simulink model "modelrevfinalPOSITIONcontrol"  (R2017b)
settings: Solver=VariableStepAuto  StartTime=0.0  StopTime=4  RelTol=1e-3
values from neighbouring files (symbols this model uses):
  D_d = 0.0034    [modelrevfinalparameters.mat]
  D_m = 0.00526687727141    [modelrevfinalparameters.mat]
  GR = 0.0526315789474    [modelrevfinalparameters.mat]
  J_l = 0.0012    [modelrevfinalparameters.mat]
  J_m = 0.0001    [modelrevfinalparameters.mat]
  k_e = 0.0064    [modelrevfinalparameters.mat]
  k_t = 0.0071    [modelrevfinalparameters.mat]
  L_a = 0.00487030359254    [modelrevfinalparameters.mat]
  m_d = 0.333333333333    [modelrevfinalparameters.mat]
  m_l = 0.333333333333    [modelrevfinalparameters.mat]
  R_a = 2.4    [modelrevfinalparameters.mat]
libraries: simulink x1
settings Model: Creator=Yusuf  LastModifiedBy=Yusuf

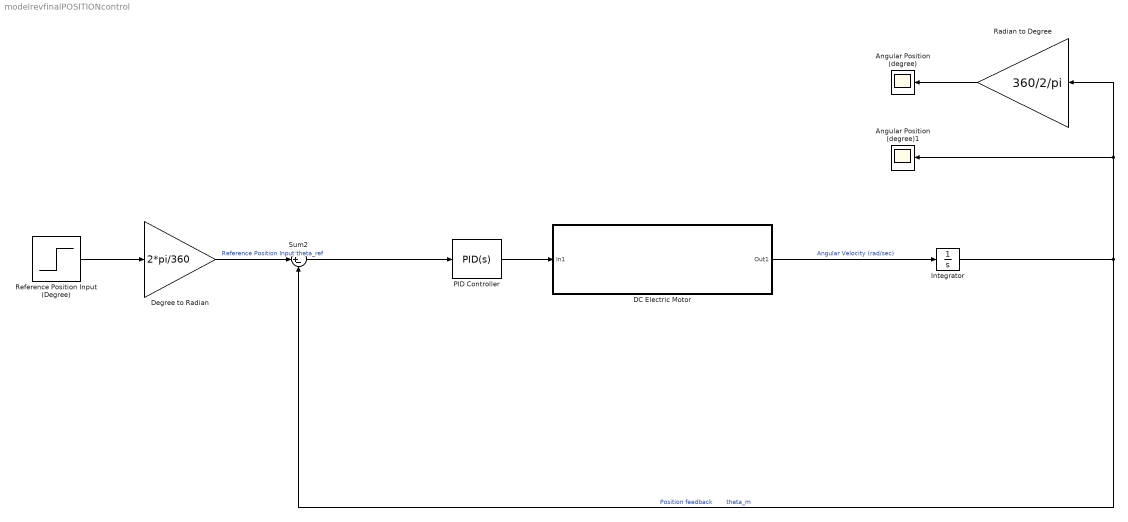
== system modelrevfinalPOSITIONcontrol ==
  Angular Position (degree) : Scope
  Angular Position (degree)1 : Scope
  DC Electric Motor : Subsystem
  Degree to Radian : Gain  Gain=2*pi/360
  Integrator : Integrator
  PID Controller : simulink/Continuous/PID Controller  Controller=PID  TimeDomain=Continuous-time  SampleTime=-1  IntegratorMethod=Forward Euler  FilterMethod=Forward Euler  Form=Parallel  UseFilter=on  ControllerParametersSource=internal  P=1.5  I=0  D=0  N=100  InitialConditionSource=internal  InitialConditionForIntegrator=0  InitialConditionForFilter=0  ExternalReset=none  LimitOutput=off  UpperSaturationLimit=inf  LowerSaturationLimit=-inf  LinearizeAsGain=on  AntiWindupMode=none  Kb=1  TrackingMode=off  Kt=1  PParamMin=[]  PParamMax=[]  IParamMin=[]  IParamMax=[]  DParamMin=[]  DParamMax=[]  NParamMin=[]  NParamMax=[]  KbParamMin=[]  KbParamMax=[]  KtParamMin=[]  KtParamMax=[]  POutMin=[]  POutMax=[]  IOutMin=[]  IOutMax=[]  DOutMin=[]  DOutMax=[]  NOutMin=[]  NOutMax=[]  KbOutMin=[]  KbOutMax=[]  KtOutMin=[]  KtOutMax=[]  IntegratorOutMin=[]  IntegratorOutMax=[]  FilterOutMin=[]  FilterOutMax=[]  SumOutMin=[]  SumOutMax=[]  SumI1OutMin=[]  SumI1OutMax=[]  SumI2OutMin=[]  SumI2OutMax=[]  SumI3OutMin=[]  SumI3OutMax=[]  SumDOutMin=[]  SumDOutMax=[]  SaturationOutMin=[]  SaturationOutMax=[]  IntegratorContinuousStateAttributes=''  IntegratorStateMustResolveToSignalObject=off  IntegratorRTWStateStorageClass=Auto  FilterContinuousStateAttributes=''  FilterStateMustResolveToSignalObject=off  FilterRTWStateStorageClass=Auto  DifferentiatorICPrevScaledInput=0  DifferentiatorOutMin=[]  DifferentiatorOutMax=[]  InitialConditionSetting=State (most efficient)  FilterDiffOutCoefMin=[]  FilterDiffOutCoefMax=[]  SumDenOutMin=[]  SumDenOutMax=[]  SumNumOutMin=[]  SumNumOutMax=[]  ReciprocalOutMin=[]  ReciprocalOutMax=[]  DivideOutMin=[]  DivideOutMax=[]  TunerSelectOption=Transfer Function Based (PID Tuner App)
  Radian to Degree : Gain  Gain=360/2/pi
  Reference Position Input (Degree) : Step  Time=0  Before=200  After=200  SampleTime=0
  Sum2 : Sum  Inputs=|+-
  wires:
  Integrator/1 -> Sum2/2, Angular Position (degree)1/1, Radian to Degree/1  "Position feedback       theta_m"
  Sum2/1 -> PID Controller/1
  DC Electric Motor/1(Out1) -> Integrator/1  "Angular Velocity (rad/sec)"
  Radian to Degree/1 -> Angular Position (degree)/1
  PID Controller/1 -> DC Electric Motor/1(In1)
  Degree to Radian/1 -> Sum2/1  "Reference Position Input theta_ref"
  Reference Position Input (Degree)/1 -> Degree to Radian/1

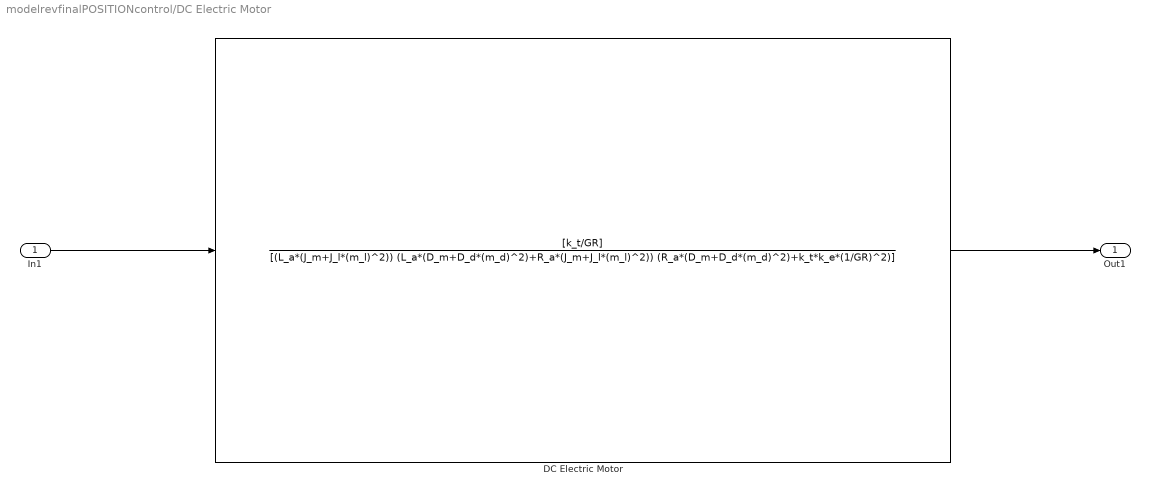
== system modelrevfinalPOSITIONcontrol/DC Electric Motor ==
  In1 : Inport
  DC Electric Motor : TransferFcn  Numerator=[k_t/GR]  Denominator=[(L_a*(J_m+J_l*(m_l)^2)) (L_a*(D_m+D_d*(m_d)^2)+R_a*(J_m+J_l*(m_l)^2)) (R_a*(D_m+D_d*(m_d)^2)+k_t*k_e*(1/GR)^2)]
  Out1 : Outport
  wires:
  In1/1 -> DC Electric Motor/1
  DC Electric Motor/1 -> Out1/1
